simulink model "MMS_ESC_B_self_driving"  (R2019b)
settings: Solver=ode45  StartTime=par.sym.TStart  StopTime=par.sym.TStop  MaxStep=par.sym.max_dt  RelTol=1e-3  EnableMultiTasking=on
undefined symbols (not defined in the file): b, B_0, eta_B, K, k, lambda_B, m, m1_B0, m2_B0, N_delay, par, Q1_B0, Q2_B0, sigma, T_tran, w_L, w_wav
libraries: simulink x1
settings Model: Creator=Vitù  LastModifiedBy=User
settings DataIOCC: SaveFormat=Array  SaveOutput=off  SignalLogging=off  DSMLogging=off  ReturnWorkspaceOutputs=off  TimeSaveName=TIME  OutputSaveName=Yout  OutputOption=SpecifiedOutputTimes  OutputTimes=[par.sym.TStart:par.sym.Outputdt:par.sym.TStop]
settings OptimizationCC: ExpressionDepthLimit=2147483647  LifeSpan=inf
settings DebuggingCC: UnderspecifiedInitializationDetection=Classic  MergeDetectMultiDrivingBlocksExec=none  SolverPrmCheckMsg=warning  AllowSymbolicDim=off  StateNameClashWarn=warning  SFUnexpectedBacktrackingDiag=warning  SFNoUnconditionalDefaultTransitionDiag=warning  SFExecutionAtInitializationDiag=none  ArithmeticOperatorsInVariantConditions=warning
settings HardwareCC: ProdBitPerPointer=32  ProdBitPerSizeT=32  ProdBitPerPtrDiffT=32  ProdLargestAtomicFloat=None  ProdIntDivRoundTo=Undefined  ProdEndianess=Unspecified  ProdWordSize=32  ProdHWDeviceType=32-bit Generic
settings ModelReferenceCC: PropagateSignalLabelsOutOfModel=off
settings SFSimCC: SimUseLocalCustomCode=off  CustomCodeUndefinedFunction=UseInterfaceOnly
settings RTWCC: RTWUseLocalCustomCode=off
settings CodeAppCC: StateflowObjectComments=on
settings GRTTargetCC: TargetLangStandard=C89/C90 (ANSI)  GeneratePreprocessorConditionals=Disable all
settings ConfigComp: CovMetricSettings=dw  CovHtmlReporting=on  CovSaveCumulativeToWorkspaceVar=on  CovSaveSingleToWorkspaceVar=on  CovExternalEMLEnable=off  CovSFcnEnable=off
settings SimscapeCC: SimscapeNormalizeSystem=off
settings ConfigurationSet: Description=SimMechanics 2G

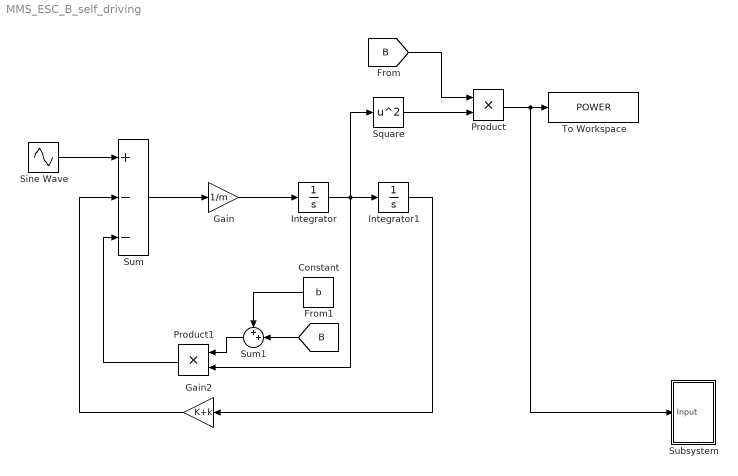
== system MMS_ESC_B_self_driving ==
  Constant : Constant  Value=b
  Gain : Gain  Gain=1/m
  Gain2 : Gain  Gain=K+k
  Integrator : Integrator
  Integrator1 : Integrator
  Product : Product
  Product1 : Product
  Sine Wave : Sin  Amplitude=par.H  Frequency=w_wav  SampleTime=0
  Square : Math  Operator=square  SignedPower=off  SaturateOnIntegerOverflow=on
  Subsystem : Subsystem
  Sum : Sum  Inputs=+--
  Sum1 : Sum  Inputs=++|
  To Workspace : ToWorkspace  VariableName=POWER  SampleTime=-1
  wires:
  Integrator1/1 -> Gain2/1
  Product/1 -> Subsystem/1(Input), To Workspace/1
  Product1/1 -> Sum/3
  Gain/1 -> Integrator/1
  Square/1 -> Product/2
  Sum/1 -> Gain/1
  Integrator/1 -> Product1/2, Square/1, Integrator1/1
  Gain2/1 -> Sum/2
  Sine Wave/1 -> Sum/1
  [B] -> Product/1
  [B] -> Sum1/2
  Sum1/1 -> Product1/1
  Constant/1 -> Sum1/1

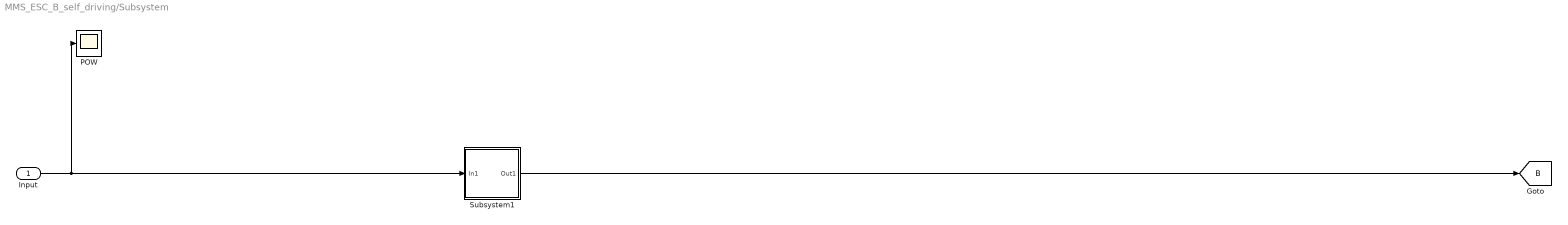
== system MMS_ESC_B_self_driving/Subsystem ==
  Input : Inport
  POW : Scope
  Subsystem1 : Subsystem
  tag scope: B=global
  wires:
  Input/1 -> Subsystem1/1(In1), POW/1
  Subsystem1/1(Out1) -> [B]

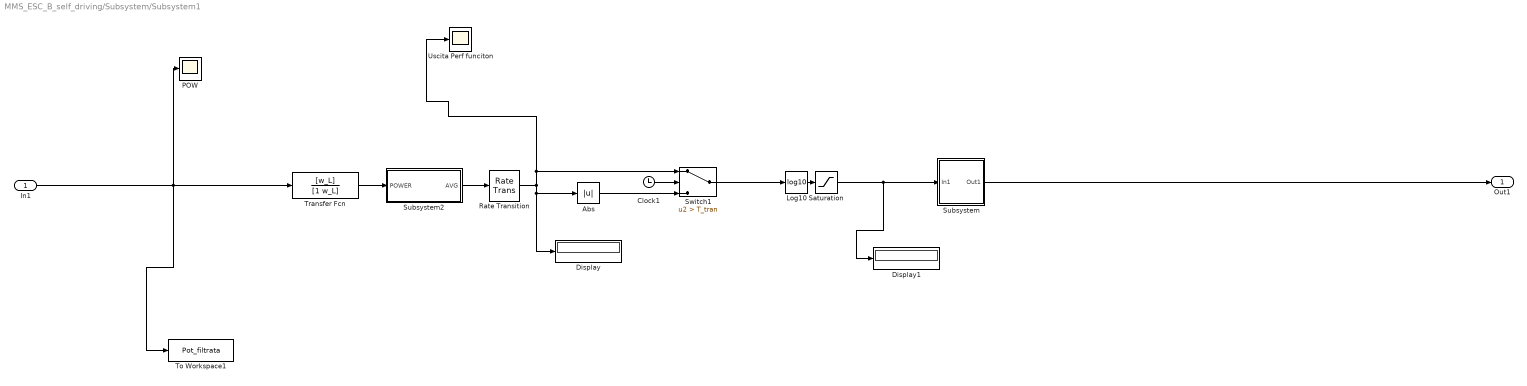
== system MMS_ESC_B_self_driving/Subsystem/Subsystem1 ==
  In1 : Inport
  Abs : Abs
  Clock1 : Clock
  Display : Display
  Display1 : Display
  Log10 : Math  Operator=log10  SignedPower=off  SaturateOnIntegerOverflow=on
  POW : Scope
  Rate Transition : RateTransition
  Saturation : Saturate  UpperLimit=inf  LowerLimit=-20
  Subsystem : Subsystem
  Subsystem2 : Subsystem
  Switch1 : Switch  Criteria=u2 > Threshold  Threshold=T_tran
  To Workspace1 : ToWorkspace  VariableName=Pot_filtrata  SampleTime=-1
  Transfer Fcn : TransferFcn  Numerator=[w_L]  Denominator=[1 w_L]
  Uscita Perf funciton : Scope
  Out1 : Outport
  wires:
  Log10/1 -> Saturation/1
  Rate Transition/1 -> Uscita Perf funciton/1, Switch1/1, Display/1, Abs/1
  Subsystem2/1(AVG) -> Rate Transition/1
  Saturation/1 -> Display1/1, Subsystem/1(In1)
  Switch1/1 -> Log10/1
  In1/1 -> To Workspace1/1, Transfer Fcn/1, POW/1
  Transfer Fcn/1 -> Subsystem2/1(POWER)
  Abs/1 -> Switch1/3
  Clock1/1 -> Switch1/2
  Subsystem/1(Out1) -> Out1/1

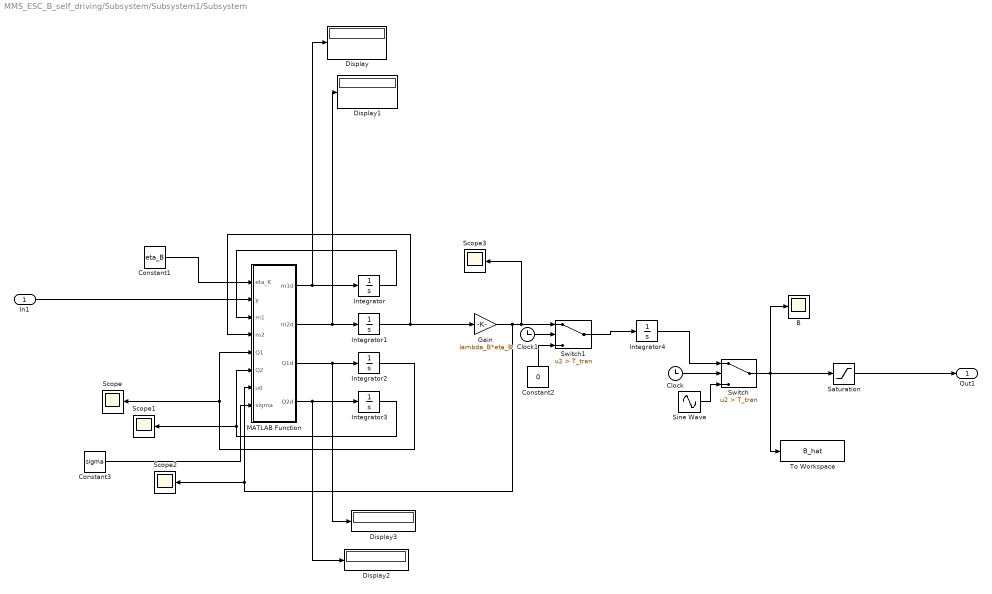
== system MMS_ESC_B_self_driving/Subsystem/Subsystem1/Subsystem ==
  In1 : Inport
  B : Scope
  Clock : Clock
  Clock1 : Clock
  Constant1 : Constant  Value=eta_B
  Constant2 : Constant  Value=0
  Constant3 : Constant  Value=sigma
  Display{,1..3} (4 alike) : Display
  Gain : Gain  Gain=lambda_B*eta_B
  Integrator : Integrator  InitialCondition=m1_B0
  Integrator1 : Integrator  InitialCondition=m2_B0
  Integrator2 : Integrator  InitialCondition=Q1_B0
  Integrator3 : Integrator  InitialCondition=Q2_B0
  Integrator4 : Integrator  InitialCondition=B_0
  MATLAB Function : MATLAB Function  TreatAsAtomicUnit=on
  Saturation : Saturate  UpperLimit=inf  LowerLimit=-b
  Scope{,1..3} (4 alike) : Scope
  Sine Wave : Sin  Bias=B_0  SampleTime=0
  Switch : Switch  Criteria=u2 > Threshold  Threshold=T_tran
  Switch1 : Switch  Criteria=u2 > Threshold  Threshold=T_tran
  To Workspace : ToWorkspace  VariableName=B_hat  SampleTime=-1
  Out1 : Outport
  wires:
  Switch/1 -> Saturation/1, To Workspace/1, B/1
  Integrator2/1 -> MATLAB Function/5(Q1), Scope/1
  Constant2/1 -> Switch1/3
  Gain/1 -> Scope3/1, Switch1/1, MATLAB Function/7(ud), Scope2/1
  Integrator1/1 -> Gain/1, MATLAB Function/4(m2)
  MATLAB Function/4(Q2d) -> Display2/1, Integrator3/1
  Integrator/1 -> MATLAB Function/3(m1)
  In1/1 -> MATLAB Function/2(y)
  Switch1/1 -> Integrator4/1
  MATLAB Function/1(m1d) -> Display/1, Integrator/1
  Integrator3/1 -> MATLAB Function/6(Q2), Scope1/1
  Sine Wave/1 -> Switch/3
  MATLAB Function/2(m2d) -> Display1/1, Integrator1/1
  Clock1/1 -> Switch1/2
  MATLAB Function/3(Q1d) -> Display3/1, Integrator2/1
  Constant1/1 -> MATLAB Function/1(eta_K)
  Constant3/1 -> MATLAB Function/8(sigma)
  Integrator4/1 -> Switch/1
  Clock/1 -> Switch/2
  Saturation/1 -> Out1/1

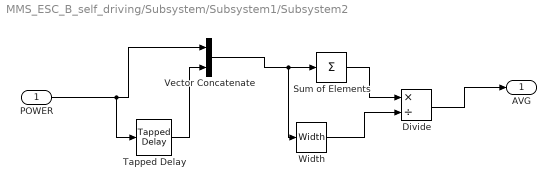
== system MMS_ESC_B_self_driving/Subsystem/Subsystem1/Subsystem2 ==
  POWER : Inport
  Divide : Product  Inputs=*/
  Sum of Elements : Sum  Inputs=+
  Tapped Delay : simulink/Discrete/Tapped Delay  vinit=0  samptime=-1  NumDelays=N_delay  DelayOrder=Oldest  includeCurrent=off
  Vector Concatenate : Concatenate
  Width : Width
  AVG : Outport
  wires:
  POWER/1 -> Tapped Delay/1, Vector Concatenate/1
  Tapped Delay/1 -> Vector Concatenate/2
  Vector Concatenate/1 -> Width/1, Sum of Elements/1
  Sum of Elements/1 -> Divide/1
  Width/1 -> Divide/2
  Divide/1 -> AVG/1

== matlab function MMS_ESC_B_self_driving/Subsystem/Subsystem1/Subsystem/MATLAB Function ==
  data: eta_K input; m1d output; y input; m1 input; m2 input; Q1 input; Q2 input; ud input; m2d output; Q1d output; Q2d output; sigma input
function [m1d,m2d,Q1d,Q2d] = SDK(eta_K,y,m1,m2,Q1,Q2,ud,sigma)
m1d = eta_K*(y-m1);
m2d = eta_K*Q1*Q2*(y-m1-Q1*m2)-sigma*eta_K*Q2*m2;
Q1d = -eta_K*Q1 + ud;
Q2d = eta_K*Q2 -eta_K*(Q1*Q2)^2-sigma*eta_K*Q2^2;
